simulink model "Nghich_luu"  (R2019a)
settings: Solver=VariableStepAuto  StartTime=0.0  StopTime=10.0  RelTol=1e-3
libraries: powerlib x13, powerlib_meascontrol x2
settings Model: Creator=Admin  LastModifiedBy=Admin

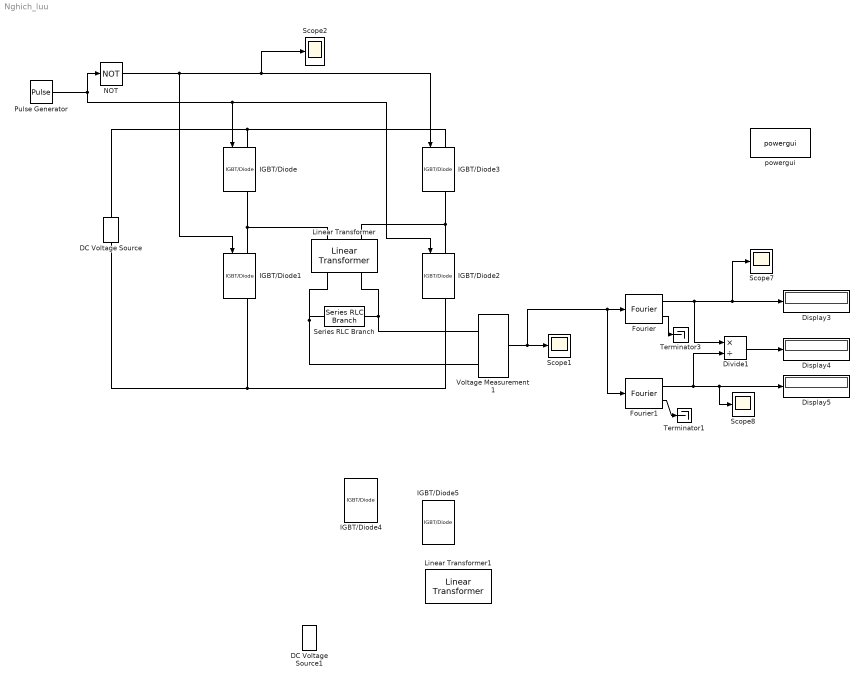
== system Nghich_luu ==
  DC Voltage Source : powerlib/Electrical Sources/DC Voltage Source  Amplitude=12  Measurements=None
      settings: SourceProductName=Simscape Electrical
  DC Voltage Source1 : powerlib/Electrical Sources/DC Voltage Source  Amplitude=12  Measurements=None
      settings: SourceProductName=Simscape Electrical
  Display3 : Display
  Display4 : Display
  Display5 : Display
  Divide1 : Product  Inputs=*/
  Fourier : powerlib_meascontrol/Measurements/Fourier  Freq=50  n=1  InInit=[0, 0]  Ts=0
      settings: SourceProductName=Simscape Electrical
  Fourier1 : powerlib_meascontrol/Measurements/Fourier  Freq=50  n=0  InInit=[0, 0]  Ts=0
      settings: SourceProductName=Simscape Electrical
  IGBT/Diode{,1..5} (6 alike) : powerlib/Power Electronics/IGBT//Diode  Ron=1e-3  Rs=1e5  Cs=inf  Measurements=on
      settings: SourceProductName=Simscape Electrical
  Linear Transformer : powerlib/Elements/Linear Transformer  UNITS=SI  NominalPower=[ 60 50 ]  winding1=[120 0 0]  winding2=[20 0.03 0.02]  ThreeWindings=off  winding3=[20 0.03 0.02]  RmLm=[Inf Inf]  Measurements=None  DataType=on
      settings: SourceProductName=Simscape Electrical
  Linear Transformer1 : powerlib/Elements/Linear Transformer  UNITS=SI  NominalPower=[ 60 50 ]  winding1=[120 0 0]  winding2=[20 0.03 0.02]  ThreeWindings=off  winding3=[20 0.03 0.02]  RmLm=[Inf Inf]  Measurements=None  DataType=on
      settings: SourceProductName=Simscape Electrical
  NOT : Logic  Operator=NOT  IconShape=distinctive  AllPortsSameDT=off  OutDataTypeStr=boolean
  Pulse Generator : DiscretePulseGenerator  PulseType=Time based  Period=0.002  PulseWidth=5
  Scope{1..2,7..8} (4 alike) : Scope
  Series RLC Branch : powerlib/Elements/Series RLC Branch  LConnTagsString=__new0  RConnTagsString=__new0  BranchType=R  Resistance=10  Inductance=1e-3  SetiL0=off  InitialCurrent=0  Capacitance=1e-6  Setx0=off  InitialVoltage=0  Measurements=None
      settings: SourceProductName=Simscape Electrical
  Terminator1 : Terminator
  Terminator3 : Terminator
  Voltage Measurement1 : powerlib/Measurements/Voltage Measurement  PhasorSimulation=off  OutputType=Complex  PSBequivalent=0
      settings: SourceProductName=Simscape Electrical
  powergui : powerlib/powergui  Priority=1  SimulationMode=Continuous  SampleTime=50e-6  frequency=60  Iterations=50  frequencyindice=0  Pbase=100e6  ErrMax=1e-4  UnitsV=kV  UnitsW=MW  buscounter=0  FunctionMessages=off  echomessages=off  EnableUseOfTLC=off  CurrentSourceSwitches=off  DisableSnubberDevices=off  DisableRonSwitches=off  DisableVfSwitches=off  DisplayEquations=off  AutomaticDiscreteSolvers=off  SolverType=Tustin/Backward Euler (TBE)  Interpol=off  ExternalGateDelay=off  methode=off  Ts=100  x0status=blocks  SPID=on  SwTol=0  HookPort=off  NonlinearTolerance=0  nMaxIteration=15  ContinueOnMaxIteration=off  RestoreLinks=warning  ResistiveCurrentMeasurement=off  Frange=[0:2:500]  Ylog=off  Xlog=on  ShowGrid=off  save=off  variable=ZData  structure=0  ZoomFFT=off  StartTime=0.0  cycles=1  DisplayStyle=1  fundamental=60  FreqAxis=off  MaxFrequency=1000  frequencyindicesteady=1  RmsSteady=1  display=off
      settings: SourceProductName=Simscape Electrical
  wires:
  Pulse Generator/1 -> NOT/1, IGBT/Diode2/1, IGBT/Diode/1
  NOT/1 -> Scope2/1, IGBT/Diode3/1, IGBT/Diode1/1
  Fourier/1 -> Divide1/1, Scope7/1, Display3/1
  Fourier1/1 -> Scope8/1, Display5/1, Divide1/2
  Fourier/2 -> Terminator3/1
  Voltage Measurement1/1 -> Scope1/1, Fourier1/1, Fourier/1
  Fourier1/2 -> Terminator1/1
  Divide1/1 -> Display4/1
  connections:
  Voltage Measurement1/LConn2 -- Linear Transformer/RConn2 -- Series RLC Branch/LConn1
  Voltage Measurement1/LConn1 -- Linear Transformer/RConn1 -- Series RLC Branch/RConn1
  IGBT/Diode/LConn1 -- IGBT/Diode3/LConn1 -- DC Voltage Source/RConn1
  IGBT/Diode/RConn1 -- Linear Transformer/LConn2 -- IGBT/Diode1/LConn1
  IGBT/Diode3/RConn1 -- Linear Transformer/LConn1 -- IGBT/Diode2/LConn1
  IGBT/Diode1/RConn1 -- DC Voltage Source/LConn1 -- IGBT/Diode2/RConn1
